simulink model "Conventional"  (R2019b)
settings: Solver=VariableStepAuto  StartTime=0.0  StopTime=867  RelTol=1e-3
libraries: qss_tb_library x6
settings Model: Creator=badk  LastModifiedBy=badk

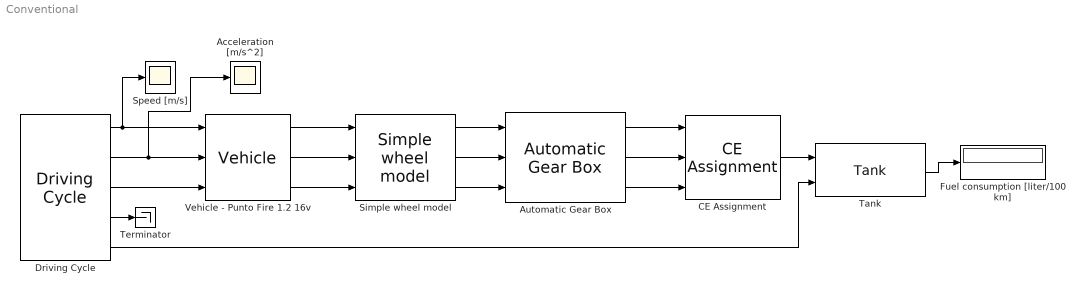
== system Conventional ==
  Acceleration [m/s^2] : Scope
  Automatic Gear Box : qss_tb_library/Gear System/Automatic Gear Box  Tag=transmission  nog=5  i=[3.909 2.158 2.158 1.121 0.921]  i_diff=4.071  gearon=[10 25 40 70]  gearoff=[2 15 30 50]  d=0.5842  e_GT=0.98  P_GT0=300  w_wheel_min=1
  CE Assignment : qss_tb_library/Energy Converter/CE Assignment  Tag=combustion engine  engine_type=Gasoline  P_ice=70  ENABLE_FUEL_CUTOFF=off
  Driving Cycle : qss_tb_library/Driving Cycle/Driving Cycle  Tag=cycle  cyclename1=City_II  stepsize=1  autostop=on
  "Fuel consumption [liter/100 km] " : Display
  Simple wheel model : qss_tb_library/Vehicle/Simple wheel model  Tag=simple transmission  d_wheel=0.5842
  Speed [m/s] : Scope
  Tank : qss_tb_library/Energy Source/Tank  Tag=tank  fuel=Gasoline  flag_cold_start=on
  Terminator : Terminator
  Vehicle - Punto Fire 1.2 16v : qss_tb_library/Vehicle/Vehicle  Tag=vehicle  m_f=936  A_f=(1.48*1.66)  cw=0.31  mu=0.012  k_inertia=4
  wires:
  Vehicle - Punto Fire 1.2 16v/1 -> Simple wheel model/1
  Vehicle - Punto Fire 1.2 16v/2 -> Simple wheel model/2
  Vehicle - Punto Fire 1.2 16v/3 -> Simple wheel model/3
  Driving Cycle/1 -> Vehicle - Punto Fire 1.2 16v/1, Speed [m/s]/1
  Driving Cycle/2 -> Acceleration [m/s^2]/1, Vehicle - Punto Fire 1.2 16v/2
  Driving Cycle/3 -> Vehicle - Punto Fire 1.2 16v/3
  Simple wheel model/1 -> Automatic Gear Box/1
  Simple wheel model/2 -> Automatic Gear Box/2
  Simple wheel model/3 -> Automatic Gear Box/3
  Automatic Gear Box/2 -> CE Assignment/2
  Automatic Gear Box/1 -> CE Assignment/1
  Automatic Gear Box/3 -> CE Assignment/3
  Tank/1 -> "Fuel consumption [liter/100 km] "/1
  CE Assignment/1 -> Tank/1
  Driving Cycle/5 -> Tank/2
  Driving Cycle/4 -> Terminator/1
